simulink model "dsp_vad"  (Simulink 8.1)
settings: Solver=VariableStepDiscrete  StartTime=0.0  StopTime=count  RelTol=1e-3
PreLoadFcn:
  | % Run the setup script when the model is opened
  | setup_dsp_vad;
InitFcn:
  | % Run the setup script again just before the
  | % model is run, so that any updates made
  | % after opening are applied.
  | setup_dsp_vad;
  | %% DSPBuilder Start
  | alt_dspbuilder_update_model(bdroot)
  | %% DSPBuilder End
StartFcn:
  | %% DSPBuilder Start
  | alt_dspbuilder_hdlimport_prepare_for_simulation(bdroot)
  | %% DSPBuilder End
values from neighbouring files (symbols this model uses):
  FS = 512    [setup_dsp_vad.m]
undefined symbols (not defined in the file or in its folder): AdvDSPBDMemDisplay, dpoly, dspba, dspba_ChannelInVis, dspba_ChannelOutVis, dspba_internal_get_channel_ports, evalAionMaskParam, pow, primtype, SF, UseDontCare, value, x, y
libraries: DSPBAPrim x267, DSPBAControl x11, DspbAdvFftLibrary x10, DSPBAModelBus x7, DSPBABase x4, simulink x3, DSPBAVectorUtil x2, DSPBAUtilities x1
(part 1 of 4)
Description:
  | DSP Builder Advanced Template for Template Design implementing Primitive Subsystems
settings Model: Creator=mjervis  LastModifiedBy=AliReza
settings DebuggingCC: InheritedTsInSrcMsg=none  IntegerOverflowMsg=none
settings ConfigurationSet: Description=SimMechanics 2G

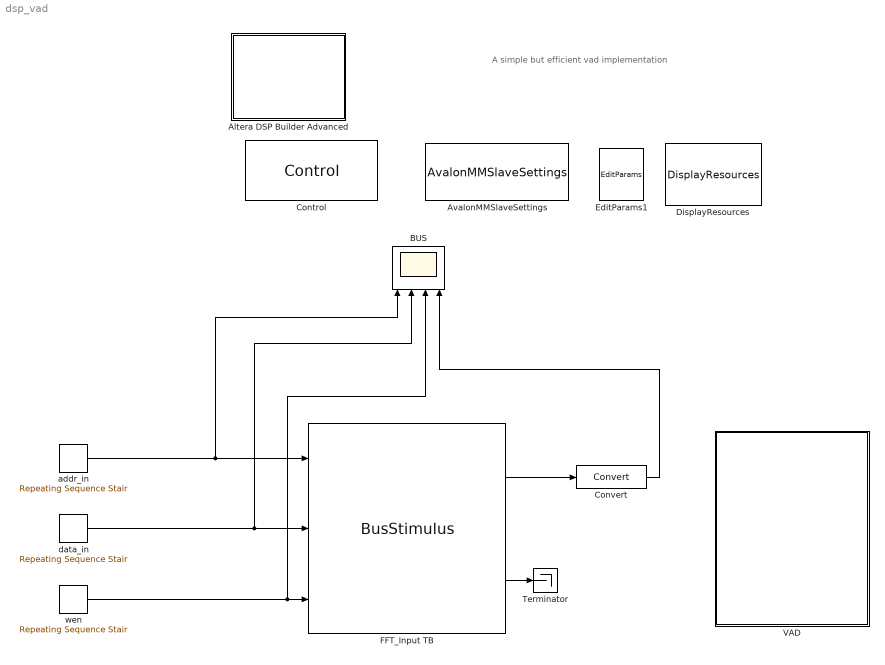
== system dsp_vad ==
  note: A simple but efficient vad implementation
  Altera DSP Builder Advanced : Subsystem  mask(DSP Builder Advanced Blockset Ignored Block){}
      settings: OpenFcn=web('http://www.altera.com', '-new');
      mask Display: image(imread('intellogo.tif'));
  AvalonMMSlaveSettings : DSPBABase/AvalonMMSlaveSettings
  BUS : Scope  NumInputPorts=4
      settings: ShowLegends=on  TimeRange=92.02958093676716  YMin=0~0~1~-1  YMax=1~1~1~1  MaxDataPoints=12290  SampleTime=auto
  "Control " : DSPBABase/Control  generate=on  language=VHDL  destination=./rtl  make_full_path=off  path_is_relative=on  autotestbench=on  signaldepth=2  coveragetestbench=off  logs=off  spacewidth=2  spacenum=1  addrwidth=10  datawidth=16  dataendian=Big Endian  hierarchicalnames=on  ramThresholdBits=-1  distRamThresholdBits=-1  mlabThresholdBits=-1  hardMultiplierThresholdLuts=-1  version=20090407  errorOnChanMismatch=1  errorOnGPIOMismatch=0  importModelsimResults=0  cycleAccurate=off  reinterpretCastMult=off  paramFile=dsp_vad_params.xml
  Convert : DSPBAPrim/Convert  primtype=convert  nInputs=1  nOutputs=1  omode=single  otype=sfix(16)  scale=2^-15  rndmethod=Biased  factor=1  satmethod=None  shift_vec=[0 1 2 -1]  value=round([0:255]/17)  inPortNames=[' '; ' ';]  outPortNames=[' '; 'c']  dspbaimage=dspba_prim.jpg  text=fprintf('convert');  style=Optimised  visibilities=8+64+256+2^17  clipdetect=off  floatPrecision=float32_m23  advOptions=[]  version=20130211
  DisplayResources : DSPBAUtilities/DisplayResources  mults=0  luts=0  memorybits=0
  EditParams1 : DSPBABase/EditParams  version=20090407
  FFT_Input TB : DSPBAModelBus/BusStimulus  SampleTime=-1  version=20140122  hasreaden=off
  Terminator : Terminator
  VAD : Subsystem
  addr_in : simulink/Sources/Repeating Sequence Stair  OutValues=dspb_vad.bus_addr_in  tsamp=1  OutMin=[]  OutMax=[]  OutDataTypeStr=fixdt(0,3)  OutputDataTypeScalingMode=Specify via dialog  OutDataType=fixdt(0,3)  ConRadixGroup=Best Precision: Vector-wise  OutScaling=[]
  data_in : simulink/Sources/Repeating Sequence Stair  OutValues=dspb_vad.bus_data_in  tsamp=1  OutMin=[]  OutMax=[]  OutDataTypeStr=single  OutputDataTypeScalingMode=single  OutDataType=fixdt(0,3)  ConRadixGroup=Best Precision: Vector-wise  OutScaling=[]
  wen : simulink/Sources/Repeating Sequence Stair  OutValues=dspb_vad.bus_wen  tsamp=1  OutMin=[]  OutMax=[]  OutDataTypeStr=fixdt('boolean')  OutputDataTypeScalingMode=Specify via dialog  OutDataType=fixdt('boolean')  ConRadixGroup=Best Precision: Vector-wise  OutScaling=[]
  wires:
  FFT_Input TB/2 -> Terminator/1
  addr_in/1 -> BUS/1, FFT_Input TB/1
  FFT_Input TB/1 -> Convert/1
  wen/1 -> BUS/3, FFT_Input TB/3
  Convert/1 -> BUS/4
  data_in/1 -> BUS/2, FFT_Input TB/2

== system dsp_vad/Altera DSP Builder Advanced ==

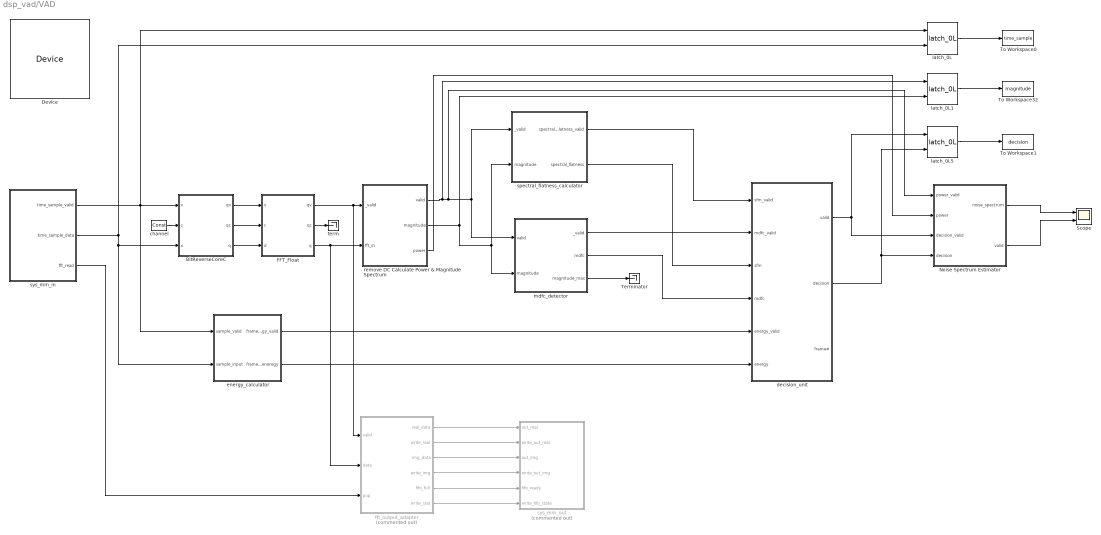
== system dsp_vad/VAD ==
  BitReverseCoreC : Subsystem  AncestorBlock=DspbAdvFftLibrary/Radix2/BitReverseCoreC  Opaque=on  mask(DSP Builder Advanced FFT Blockset){N=512, subchannels=1}
      mask prompts: N "FFT Size"; subchannels "Number of subchannels (must be a power of 2)"
      mask help: Performs bit reversal of incoming FFT frames.
      mask init:
      | block = gcb;
      | 
      | % Check that we have a legal size
      | M = ceil(log2(N));
      | if not(N == 2^M)
      |     error('%s: %d is not a power of 2', block, N);
      | end
      | 
      | % Check that we have a legal number os subchannels
      | subchannelbits = ceil(log2(subchannels));
      | if not(subchannels == 2^subchannelbits)
      |     error('%s: subchannels count %d is not a power of 2', block, N);
      | end
      | 
      | % The permutation reverses the order of the address bits
      | bitrevperm = [M-1:-1:0];
      | 
      | % Prefix permutaion with unchanging subchannel bits
      | bitrevperm = [0:subchannelbits-1,bitrevperm+subchannelbits];
      | 
      | if 1 < subchannels
      |     subchannelString = sprintf('%d subchannels',subchannels);
      | else
      |     subchannelString = '';
      | end
      mask Help: helpview(dspba.GetHelp('BitReverseCore'));
      mask Display:
      | color('w');
      | image('dspba_fft.jpg');
      | port_label('input',1,'v');
      | port_label('input',2,'c');
      | port_label('input',3,'x');
      | port_label('output',1,'qv');
      | port_label('output',2,'qc');
      | port_label('output',3,'q');
      | text(0.45,0.7,'Bit');
      | text(0.35,0.6,'Reverse');
      | text(0.40,0.5, sprintf('%d',N));
      | text(0.5,0.1,sprintf('Radix 2'),'texmode','on');
      | text(0.20,0.35,subchannelString);
  Device : DSPBABase/Device  family=Cyclone V  stratix4device=Stratix IV E  hardcopy4device=HardCopy IV E  stratix5device=Stratix V GX  device=AUTO  speed=1  stratixSpeed=-5  stratix2Speed=-3  stratix3Speed=-2  stratix4gxSpeed=-2  stratix4gtSpeed=-1  cyclone2Speed=-6  cyclone3Speed=-7  arria2Speed=-4  cyclone4eSpeed=-8  stratix5Speed=-3  arria5Speed=-4  arriaSpeed=-6  cyclone3lsSpeed=-7  cyclone5Speed=-6  arria2gzSpeed=-3  nightFurySpeed=-2  ecp2Speed=-7  hardcopycompat=off  version=20140217  max10flashmode=off  max10nomeminit=off
  FFT_Float : Subsystem  AncestorBlock=DspbAdvFftLibrary/Floating Point/FP_FFT  Opaque=on  mask{FFTstring=FFT, orderString=Bit Reversed, N=9, twiddle_type=single, faithful=false}
      mask prompts: FFTstring "FFT type"; orderString "Input Order"; N "N, where the (I)FFT has size 2^N"; twiddle_type "Data type"; faithful "Use faithful rounding"
      mask init:
      | block = gcb;
      | 
      | br_in = strcmp(orderString,'Bit Reversed');
      | IFFT = strcmp(FFTstring,'IFFT');
      | 
      | % Assume input type is the same as the twiddle type
      | data_type = dspba.namedVPFloat(twiddle_type);
      | type_strings = ...
      |     dspba.fft.full_wordgrowth(...
      |         true, false, N, data_type, data_type);
      | 
      | if br_in
      |     directionString = 'BR->NAT';
      | else
      |     directionString = 'NAT->BR';
      | end
      mask Help: helpview(dspba.GetHelp('fft'));
      mask TypeOptions FFTstring: FFT | IFFT
      mask TypeOptions orderString: Bit Reversed | Natural Order
      mask TypeOptions twiddle_type: single | double | float16_m10 | float26_m17 | float32_m23 | float35_m26 | float46_m35 | float55_m44 | float64_m52
      mask Display:
      | color('w');
      | image('dspba_fft.jpg');
      | port_label('input',1,'v');
      | port_label('input',2,'c');
      | port_label('input',3,'d');
      | port_label('output',1,'qv');
      | port_label('output',2,'qc');
      | port_label('output',3,'q');
      | text(0.30,0.65,sprintf('%s Core',FFTstring));
      | text(0.45,0.55,sprintf('2^{%d}',N),'texmode','on');
      | text(0.30,0.45,directionString);
  Noise Spectrum Estimator : Subsystem
  Scope : Scope  NumInputPorts=2
      settings: YMin=0~0  YMax=0.017~1  SaveName=ScopeData2
  Terminator : Terminator
  To Workspace0 : ToWorkspace  VariableName=time_sample  SampleTime=-1
  To Workspace1 : ToWorkspace  VariableName=decision  SampleTime=-1
  To Workspace32 : ToWorkspace  VariableName=magnitude  SampleTime=-1
  channel : DSPBAPrim/Const  primtype=const  nInputs=0  nOutputs=1  omode=Inherit via back propagation  otype=zeros(1,1,uint(8))  scale=1  rndmethod=Unbiased  factor=1  satmethod=Symmetric  shift_vec=[0 1 2 -1]  value=0  inPortNames=['+'; '+';]  outPortNames=[' ']  dspbaimage=dspba_prim.jpg  text=fprintf('%s', num2str(value));  style=Optimised  visibilities=8 + 1024  floatPrecision=float32_m23  version=20120820
  decision_unit : Subsystem
  energy_calculator : Subsystem
  fft_output_adapter : Subsystem  Commented=on
  latch_0L : DSPBAControl/latch_0L
  latch_0L1 : DSPBAControl/latch_0L
  latch_0L5 : DSPBAControl/latch_0L
  mdfc_detector : Subsystem
  remove DC Calculate Power & Magnitude Spectrum : Subsystem
  spectral_flatness_calculator : Subsystem
  sys_mm_in : Subsystem
  sys_mm_out : Subsystem  Commented=on
  "term " : Terminator
  wires:
  fft_output_adapter/1(real_data) -> sys_mm_out/1(out_real)
  fft_output_adapter/2(write_real) -> sys_mm_out/2(write_out_real)
  fft_output_adapter/3(img_data) -> sys_mm_out/3(out_img)
  fft_output_adapter/4(write_img) -> sys_mm_out/4(write_out_img)
  fft_output_adapter/5(fifo_full) -> sys_mm_out/5(fifo_ready)
  fft_output_adapter/6(write_stat) -> sys_mm_out/6(write_fifo_state)
  sys_mm_in/1(time_sample_valid) -> latch_0L/1, energy_calculator/1(sample_valid), BitReverseCoreC/1(v)
  FFT_Float/1(qv) -> remove DC Calculate Power & Magnitude Spectrum/1(_valid), fft_output_adapter/1(valid)
  FFT_Float/3(q) -> remove DC Calculate Power & Magnitude Spectrum/2(fft_in), fft_output_adapter/2(data)
  BitReverseCoreC/3(q) -> FFT_Float/3(d)
  channel/1 -> BitReverseCoreC/2(c)
  FFT_Float/2(qc) -> "term "/1
  BitReverseCoreC/2(qc) -> FFT_Float/2(c)
  BitReverseCoreC/1(qv) -> FFT_Float/1(v)
  sys_mm_in/2(time_sample_data) -> energy_calculator/2(sample_input), BitReverseCoreC/3(x), latch_0L/2
  sys_mm_in/3(fft_read) -> fft_output_adapter/3(pop)
  remove DC Calculate Power & Magnitude Spectrum/1(valid) -> spectral_flatness_calculator/1(_valid), mdfc_detector/1(valid), Noise Spectrum Estimator/1(power_valid), latch_0L1/1
  mdfc_detector/3(magnitude_max) -> Terminator/1
  energy_calculator/1(frame_energy_valid) -> decision_unit/5("energy_valid ")
  energy_calculator/2(frame_eneregy) -> decision_unit/6(energy)
  mdfc_detector/2(mdfc) -> decision_unit/4(mdfc)
  spectral_flatness_calculator/2(spectral_flatness) -> decision_unit/3(sfm)
  mdfc_detector/1(_valid) -> decision_unit/2(mdfc_valid)
  spectral_flatness_calculator/1(spectral_flatness_valid) -> decision_unit/1(sfm_valid)
  latch_0L/1 -> To Workspace0/1
  decision_unit/1(valid) -> latch_0L5/1, Noise Spectrum Estimator/3(decision_valid)
  decision_unit/2(decision) -> latch_0L5/2, Noise Spectrum Estimator/4(decision)
  latch_0L1/1 -> To Workspace32/1
  latch_0L5/1 -> To Workspace1/1
  remove DC Calculate Power & Magnitude Spectrum/2(magnitude) -> latch_0L1/2, mdfc_detector/2(magnitude), spectral_flatness_calculator/2(magnitude)
  remove DC Calculate Power & Magnitude Spectrum/3(power) -> Noise Spectrum Estimator/2(power)
  Noise Spectrum Estimator/1(noise_spectrum) -> Scope/1
  Noise Spectrum Estimator/2(valid) -> Scope/2

== system dsp_vad/VAD/BitReverseCoreC ==
  note: Bit-accurate simulation used
  note: Each block of 2^N samples should
      |  use the same channel number.
      |
      | So we latch the channel number on
      |  the last valid input (first valid output)
      | of each block.
  v : Inport
  c : Inport  Port=2
  x : Inport  Port=3
  ChannelIn : DSPBAPrim/ChannelIn  primtype=channelin  nInputs=dspba_internal_get_channel_ports(gcb)  nOutputs=dspba_internal_get_channel_ports(gcb)  omode=Inherit via internal rule  otype=sfix(16)  scale=2^-15  rndmethod=Unbiased  factor=1  satmethod=Symmetric  shift_vec=[0 1 2 -1]  value=1  inPortNames=['v'; 'c'; '0'; '1'; '2'; '3'; '4'; '5'; '6'; '7'; '8'; '9'; 'a'; 'b']  outPortNames=['v'; 'c'; '0'; '1'; '2'; '3'; '4'; '5'; '6'; '7'; '8'; '9'; 'a'; 'b']  dspbaimage=dspba_prim.jpg  text=fprintf('In');  style=Optimised  dataSignals=1  foldingEnabled=off  channels=1  sampleRate=200  packetBeginPresent=off  packetBeginEnabled=off  visibilities=1024  latencyCorrection=0  scheduleOrigin=on  version=20141013
  ChannelOut : DSPBAPrim/ChannelOut  primtype=channelout  nInputs=dspba_internal_get_channel_ports(gcb)  nOutputs=dspba_internal_get_channel_ports(gcb)  omode=Inherit via internal rule  otype=sfix(16)  scale=2^-15  rndmethod=Unbiased  factor=1  satmethod=Symmetric  shift_vec=[0 1 2 -1]  value=1  inPortNames=['v'; 'c'; '0'; '1'; '2'; '3'; '4'; '5'; '6'; '7'; '8'; '9']  outPortNames=['v'; 'c'; '0'; '1'; '2'; '3'; '4'; '5'; '6'; '7'; '8'; '9']  dspbaimage=dspba_prim.jpg  text=fprintf('Out');  style=Optimised  dataSignals=1  foldingEnabled=off  channels=1  sampleRate=200  packetBeginPresent=off  packetBeginEnabled=off  visibilities=1024  latency=0  latencyCorrection=0  version=20141013
  SynthesisInfo : DSPBAPrim/SynthesisInfo  primtype=synthinfo  nInputs=0  nOutputs=0  omode=Inherit via internal rule  otype=sfix(16)  scale=2^-15  rndmethod=Truncate  factor=1  satmethod=Symmetric  shift_vec=[0 1 2 -1]  value=99  inPortNames=[' '; ' ';]  outPortNames=[' ']  dspbaimage=dspba_prim_ctrl.jpg  text=fprintf('Style=%s', style);  style=Scheduled  visibilities=32768  constraintInUse=off  constraintRelation=>  constraintLimit=2  bitAccurate=on  version=20150220
  Transpose : DspbAdvFftLibrary/Common/Transpose  perm=bitrevperm
  latch_0L : DSPBAControl/latch_0L
  qv : Outport
  qc : Outport  Port=2
  q : Outport  Port=3
  wires:
  Transpose/3 -> latch_0L/1
  Transpose/2 -> ChannelOut/3
  Transpose/1 -> ChannelOut/1
  ChannelIn/3 -> Transpose/2
  ChannelIn/1 -> Transpose/1
  ChannelIn/2 -> latch_0L/2
  latch_0L/1 -> ChannelOut/2
  ChannelOut/3 -> q/1
  ChannelOut/2 -> qc/1
  ChannelOut/1 -> qv/1
  c/1 -> ChannelIn/2
  v/1 -> ChannelIn/1
  x/1 -> ChannelIn/3

== system dsp_vad/VAD/FFT_Float ==
  note: Bit-accurate simulation used
  note: Each block of 2^N samples should use the same channel
      | and starts arriving on the output after 2^N-1 cycles.
      |
      | So we latch the channel number on
      |  the last valid input of each block.
  v : Inport
  c : Inport  Port=2
  d : Inport  Port=3
  ChannelIn : DSPBAPrim/ChannelIn  primtype=channelin  nInputs=dspba_internal_get_channel_ports(gcb)  nOutputs=dspba_internal_get_channel_ports(gcb)  omode=Inherit via internal rule  otype=sfix(16)  scale=2^-15  rndmethod=Unbiased  factor=1  satmethod=Symmetric  shift_vec=[0 1 2 -1]  value=1  inPortNames=['v'; 'c'; '0'; '1'; '2'; '3'; '4'; '5'; '6'; '7'; '8'; '9'; 'a'; 'b']  outPortNames=['v'; 'c'; '0'; '1'; '2'; '3'; '4'; '5'; '6'; '7'; '8'; '9'; 'a'; 'b']  dspbaimage=dspba_prim.jpg  text=fprintf('In');  style=Optimised  dataSignals=1  foldingEnabled=off  channels=1  sampleRate=200  packetBeginPresent=off  packetBeginEnabled=off  visibilities=dspba_ChannelInVis(gcb)  latencyCorrection=0  scheduleOrigin=on  version=20141013
  ChannelOut1 : DSPBAPrim/ChannelOut  primtype=channelout  nInputs=dspba_internal_get_channel_ports(gcb)  nOutputs=dspba_internal_get_channel_ports(gcb)  omode=Inherit via internal rule  otype=sfix(16)  scale=2^-15  rndmethod=Unbiased  factor=1  satmethod=Symmetric  shift_vec=[0 1 2 -1]  value=1  inPortNames=['v'; 'c'; '0'; '1'; '2'; '3'; '4'; '5'; '6'; '7'; '8'; '9']  outPortNames=['v'; 'c'; '0'; '1'; '2'; '3'; '4'; '5'; '6'; '7'; '8'; '9']  dspbaimage=dspba_prim.jpg  text=fprintf('Out');  style=Optimised  dataSignals=1  foldingEnabled=off  channels=1  sampleRate=200  packetBeginPresent=off  packetBeginEnabled=off  visibilities=dspba_ChannelOutVis(gcb)  latency=0  latencyCorrection=0  version=20141013
  FP FFT Light : DspbAdvFftLibrary/Common/FFT_Light  IFFT=IFFT  subchannels=1  br_in=br_in  N=N  in_type=data_type  type_strings=type_strings  faithful=faithful  wirecount=1
  SynthesisInfo : DSPBAPrim/SynthesisInfo  primtype=synthinfo  nInputs=0  nOutputs=0  omode=Inherit via internal rule  otype=sfix(16)  scale=2^-15  rndmethod=Truncate  factor=1  satmethod=Symmetric  shift_vec=[0 1 2 -1]  value=99  inPortNames=[' '; ' ';]  outPortNames=[' ']  dspbaimage=dspba_prim.jpg  text=fprintf('Style=%s', style);  style=Scheduled  visibilities=32768  constraintInUse=off  constraintRelation=>  constraintLimit=2  bitAccurate=on  version=20150220
  latch_0L : DSPBAControl/latch_0L
  qv : Outport
  qc : Outport  Port=2
  q : Outport  Port=3
  wires:
  FP FFT Light/3 -> latch_0L/1
  ChannelIn/2 -> latch_0L/2
  FP FFT Light/2 -> ChannelOut1/3
  ChannelIn/3 -> FP FFT Light/2
  v/1 -> ChannelIn/1
  d/1 -> ChannelIn/3
  c/1 -> ChannelIn/2
  ChannelIn/1 -> FP FFT Light/1
  latch_0L/1 -> ChannelOut1/2
  ChannelOut1/3 -> q/1
  ChannelOut1/1 -> qv/1
  ChannelOut1/2 -> qc/1
  FP FFT Light/1 -> ChannelOut1/1

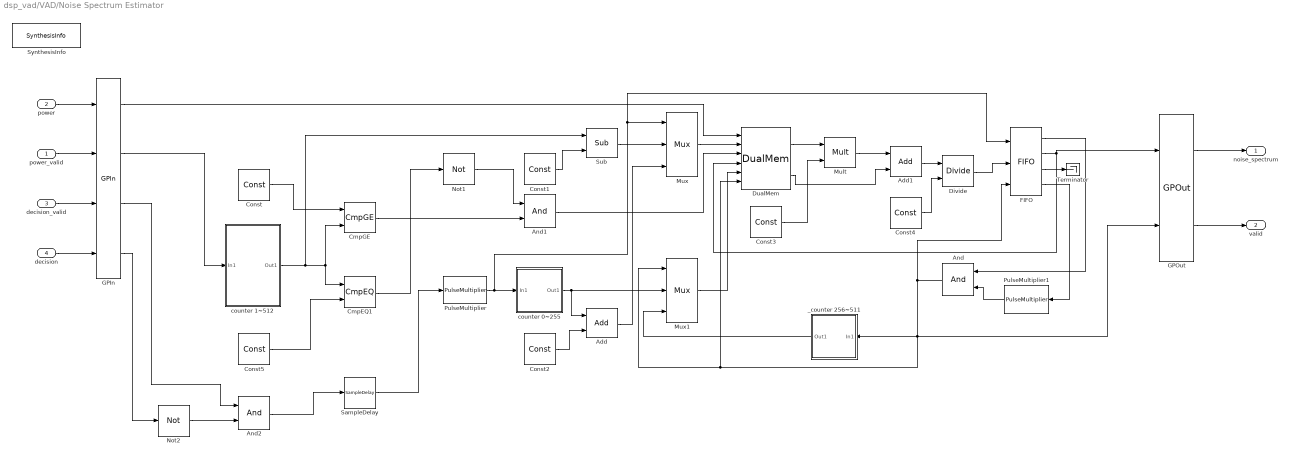
== system dsp_vad/VAD/Noise Spectrum Estimator ==
  power_valid : Inport
  power : Inport  Port=2
  decision_valid : Inport  Port=3
  decision : Inport  Port=4
  Add : DSPBAPrim/Add  primtype=add  nInputs=evalAionMaskParam(gcb,'value',1)  nOutputs=1  omode=Specify via dialog  otype=ufix(10)  scale=2^-0  rndmethod=Unbiased  factor=1  satmethod=Symmetric  shift_vec=[0 1 2 -1]  value=2  inPortNames=[' '; ' ';]  outPortNames=[' ']  dspbaimage=dspba_prim.jpg  text=fprintf('+');  style=Optimised  visibilities=1032+2^17+2^18+2^19  genFPC=off  floatRounding=correct  advOptions=[]  version=20130821
  Add1 : DSPBAPrim/Add  primtype=add  nInputs=evalAionMaskParam(gcb,'value',1)  nOutputs=1  omode=Inherit via internal rule  otype=ufix(10)  scale=2^-0  rndmethod=Unbiased  factor=1  satmethod=Symmetric  shift_vec=[0 1 2 -1]  value=2  inPortNames=[' '; ' ';]  outPortNames=[' ']  dspbaimage=dspba_prim.jpg  text=fprintf('+');  style=Optimised  visibilities=1032+2^17+2^18+2^19  genFPC=off  floatRounding=correct  advOptions=[]  version=20130821
  And : DSPBAPrim/And  primtype=and  nInputs=2  nOutputs=1  omode=Inherit via internal rule  otype=sfix(16)  scale=2^-15  rndmethod=Unbiased  factor=1  satmethod=Symmetric  shift_vec=[0 1 2 -1]  value=0  inPortNames=[' '; ' '; ' '; ' '; ' '; ' '; ' '; ' '; ' '; ' '; ' '; ' '; ' '; ' '; ' '; ' '; ]  outPortNames=[' ']  dspbaimage=dspba_prim.jpg  text=fprintf('&');  style=Optimised  visibilities=8+2  version=20090407
  And1 : DSPBAPrim/And  primtype=and  nInputs=2  nOutputs=1  omode=Inherit via internal rule  otype=sfix(16)  scale=2^-15  rndmethod=Unbiased  factor=1  satmethod=Symmetric  shift_vec=[0 1 2 -1]  value=0  inPortNames=[' '; ' '; ' '; ' '; ' '; ' '; ' '; ' '; ' '; ' '; ' '; ' '; ' '; ' '; ' '; ' '; ]  outPortNames=[' ']  dspbaimage=dspba_prim.jpg  text=fprintf('&');  style=Optimised  visibilities=8+2  version=20090407
  And2 : DSPBAPrim/And  primtype=and  nInputs=2  nOutputs=1  omode=Inherit via internal rule  otype=sfix(16)  scale=2^-15  rndmethod=Unbiased  factor=1  satmethod=Symmetric  shift_vec=[0 1 2 -1]  value=0  inPortNames=[' '; ' '; ' '; ' '; ' '; ' '; ' '; ' '; ' '; ' '; ' '; ' '; ' '; ' '; ' '; ' '; ]  outPortNames=[' ']  dspbaimage=dspba_prim.jpg  text=fprintf('&');  style=Optimised  visibilities=8+2  version=20090407
  CmpEQ1 : DSPBAPrim/CmpEQ  primtype=cmpeq  nInputs=2  nOutputs=1  omode=boolean  otype=sfix(16)  scale=2^-15  rndmethod=Unbiased  factor=1  satmethod=Symmetric  shift_vec=[0 1 2 -1]  value=0  inPortNames=[' '; ' ';]  outPortNames=[' ']  dspbaimage=dspba_prim.jpg  text=fprintf('==');  style=Optimised  visibilities=0  advOptions=[]  version=20130117
  CmpGE : DSPBAPrim/CmpGE  primtype=cmpgte  nInputs=2  nOutputs=1  omode=boolean  otype=sfix(16)  scale=2^-15  rndmethod=Unbiased  factor=1  satmethod=Symmetric  shift_vec=[0 1 2 -1]  value=0  inPortNames=['a'; 'b';]  outPortNames=[' ']  dspbaimage=dspba_prim.jpg  text=fprintf('a>=b');  style=Optimised  visibilities=0  advOptions=[]  version=20130117
  Const : DSPBAPrim/Const  primtype=const  nInputs=0  nOutputs=1  omode=Specify via dialog  otype=ufix(9)  scale=2^-0  rndmethod=Unbiased  factor=1  satmethod=Symmetric  shift_vec=[0 1 2 -1]  value=256  inPortNames=['+'; '+';]  outPortNames=[' ']  dspbaimage=dspba_prim.jpg  text=fprintf('%s', num2str(value));  style=Optimised  visibilities=8 + 1024  floatPrecision=float32_m23  version=20120820
  Const1 : DSPBAPrim/Const  primtype=const  nInputs=0  nOutputs=1  omode=Specify via dialog  otype=ufix(10)  scale=2^-0  rndmethod=Unbiased  factor=1  satmethod=Symmetric  shift_vec=[0 1 2 -1]  value=1  inPortNames=['+'; '+';]  outPortNames=[' ']  dspbaimage=dspba_prim.jpg  text=fprintf('%s', num2str(value));  style=Optimised  visibilities=8 + 1024  floatPrecision=float32_m23  version=20120820
  Const2 : DSPBAPrim/Const  primtype=const  nInputs=0  nOutputs=1  omode=Specify via dialog  otype=ufix(10)  scale=2^-0  rndmethod=Unbiased  factor=1  satmethod=Symmetric  shift_vec=[0 1 2 -1]  value=256  inPortNames=['+'; '+';]  outPortNames=[' ']  dspbaimage=dspba_prim.jpg  text=fprintf('%s', num2str(value));  style=Optimised  visibilities=8 + 1024  floatPrecision=float32_m23  version=20120820
  Const3 : DSPBAPrim/Const  primtype=const  nInputs=0  nOutputs=1  omode=single  otype=sfix(16)  scale=2^-15  rndmethod=Unbiased  factor=1  satmethod=Symmetric  shift_vec=[0 1 2 -1]  value=30  inPortNames=['+'; '+';]  outPortNames=[' ']  dspbaimage=dspba_prim.jpg  text=fprintf('%s', num2str(value));  style=Optimised  visibilities=8 + 1024  floatPrecision=float32_m23  version=20120820
  Const4 : DSPBAPrim/Const  primtype=const  nInputs=0  nOutputs=1  omode=single  otype=sfix(16)  scale=2^-15  rndmethod=Unbiased  factor=1  satmethod=Symmetric  shift_vec=[0 1 2 -1]  value=31  inPortNames=['+'; '+';]  outPortNames=[' ']  dspbaimage=dspba_prim.jpg  text=fprintf('%s', num2str(value));  style=Optimised  visibilities=8 + 1024  floatPrecision=float32_m23  version=20120820
  Const5 : DSPBAPrim/Const  primtype=const  nInputs=0  nOutputs=1  omode=Specify via dialog  otype=ufix(10)  scale=2^-0  rndmethod=Unbiased  factor=1  satmethod=Symmetric  shift_vec=[0 1 2 -1]  value=0  inPortNames=['+'; '+';]  outPortNames=[' ']  dspbaimage=dspba_prim.jpg  text=fprintf('%s', num2str(value));  style=Optimised  visibilities=8 + 1024  floatPrecision=float32_m23  version=20120820
  Divide : DSPBAPrim/Divide  primtype=divide  nInputs=2  nOutputs=1  omode=Inherit via internal rule  otype=sfix(16)  scale=2^-15  rndmethod=Unbiased  factor=1  satmethod=Symmetric  shift_vec=[0 1 2 -1]  value=round([0:255]/17)  inPortNames=[' '; ' ';]  outPortNames=[' ']  dspbaimage=dspba_prim.jpg  text=fprintf('a\n----\nb');  style=Optimised  visibilities=8+2^17+2^18  floatRounding=correct  advOptions=[]  version=20130115
  DualMem : DSPBAPrim/DualMem  primtype=dualmem  nInputs=6  nOutputs=2  omode=single  otype=sfix(16)  scale=2^-15  rndmethod=Unbiased  factor=1  satmethod=Symmetric  shift_vec=[0 1 2 -1]  value=[zeros(512, 1)]  inPortNames=['d1'; 'a1'; 'w1'; 'd2'; 'a2'; 'w2']  outPortNames=['q1'; 'q2']  dspbaimage=dspba_prim.jpg  text=fprintf('dmem%s',AdvDSPBDMemDisplay(UseDontCare));  style=Optimised  visibilities=8 + 1024 + 2^17 + 2^18  UseDontCare=on  TwinWritePorts=on  version=20141001
  FIFO : DSPBAPrim/FIFO  primtype=fifo  nInputs=3  nOutputs=4  omode=Inherit via internal rule  otype=sfix(16)  scale=2^-15  rndmethod=Unbiased  factor=1  satmethod=Symmetric  shift_vec=[0 1 2 -1]  value=[256 1 256]  inPortNames=['w'; 'd'; 'r'; 'f']  outPortNames=['v'; 'q'; 't'; 'f']  dspbaimage=dspba_prim.jpg  text=fprintf('fifo');  style=Optimised  visibilities=263168  version=20130808  user_sclr=off
  GPIn : DSPBAPrim/GPIn  primtype=gpin  nInputs=evalAionMaskParam(gcb,'value',1)  nOutputs=evalAionMaskParam(gcb,'value',1)  omode=Inherit via internal rule  otype=sfix(16)  scale=2^-15  rndmethod=Unbiased  factor=1  satmethod=Symmetric  shift_vec=[0 1 2 -1]  value=4  inPortNames=[' ' ' ' ' ' ' ' ' ' ' ' ' ' ' ' ' ' ' ' ' ' ' ' ' ' ' ' ' ' ' ' ' ' ' ' ' ' ' ' ' ' ' ' ' ' ' ' ' ' ' ' ' ' ' ' ' ' ' ' ' ' ' ' ' ' ' ' ' ']'  outPortNames=[' ' ' ' ' ' ' ' ' ' ' ' ' ' ' ' ' ' ' ' ' ' ' ' ' ' ' ' ' ' ' ' ' ' ' ' ' ' ' ' ' ' ' ' ' ' ' ' ' ' ' ' ' ' ' ' ' ' ' ' ' ' ' ' ' ' ' ' ' ']'  dspbaimage=dspba_prim.jpg  text=fprintf('GPIn');  style=Optimised  visibilities=1024  latencyCorrection=0  scheduleOrigin=on  version=20090407
  GPOut : DSPBAPrim/GPOut  primtype=gpout  nInputs=evalAionMaskParam(gcb,'value',1)  nOutputs=evalAionMaskParam(gcb,'value',1)  omode=Inherit via internal rule  otype=sfix(16)  scale=2^-15  rndmethod=Unbiased  factor=1  satmethod=Symmetric  shift_vec=[0 1 2 -1]  value=2  inPortNames=[' ' ' ' ' ' ' ' ' ' ' ' ' ' ' ' ' ' ' ' ' ' ' ' ' ' ' ' ' ' ' ' ' ' ' ' ' ' ' ' ' ' ' ' ' ' ' ' ' ' ' ' ' ' ' ' ' ' ' ' ' ' ' ' ' ' ' ' ' ']'  outPortNames=[' ' ' ' ' ' ' ' ' ' ' ' ' ' ' ' ' ' ' ' ' ' ' ' ' ' ' ' ' ' ' ' ' ' ' ' ' ' ' ' ' ' ' ' ' ' ' ' ' ' ' ' ' ' ' ' ' ' ' ' ' ' ' ' ' ' ' ' ' ']'  dspbaimage=dspba_prim.jpg  text=fprintf('GPOut');  style=Optimised  visibilities=1024  latencyCorrection=0  version=20090407
  Mult : DSPBAPrim/Mult  primtype=mult  nInputs=2  nOutputs=1  omode=Inherit via internal rule  otype=sfix(16)  scale=2^-15  rndmethod=Unbiased  factor=1  satmethod=Symmetric  shift_vec=[0 1 2 -1]  value=0  inPortNames=[' '; ' ';]  outPortNames=[' ']  dspbaimage=dspba_prim.jpg  text=fprintf('X');  style=Optimised  visibilities=8+2^18+2^19  floatPrecision=float32_m23  floatRounding=correct  advOptions=[]  version=20130115
  Mux : DSPBAPrim/Mux  primtype=mux  nInputs=evalAionMaskParam(gcb,'value',1)+1  nOutputs=1  omode=Inherit via internal rule  otype=sfix(16)  scale=2^-15  rndmethod=Unbiased  factor=1  satmethod=Symmetric  shift_vec=[0 1 2 -1]  value=2  inPortNames=['s '; 'd0'; 'd1'; 'd2'; 'd3'; 'd4'; 'd5'; 'd6'; 'd7'; 'd8'; 'd9';]  outPortNames=[' ']  dspbaimage=dspba_prim.jpg  text=fprintf('%s', primtype);  style=Optimised  visibilities=1032  version=20131025
  Mux1 : DSPBAPrim/Mux  primtype=mux  nInputs=evalAionMaskParam(gcb,'value',1)+1  nOutputs=1  omode=Inherit via internal rule  otype=sfix(16)  scale=2^-15  rndmethod=Unbiased  factor=1  satmethod=Symmetric  shift_vec=[0 1 2 -1]  value=2  inPortNames=['s '; 'd0'; 'd1'; 'd2'; 'd3'; 'd4'; 'd5'; 'd6'; 'd7'; 'd8'; 'd9';]  outPortNames=[' ']  dspbaimage=dspba_prim.jpg  text=fprintf('%s', primtype);  style=Optimised  visibilities=1032  version=20131025
  Not1 : DSPBAPrim/Not  primtype=not  nInputs=1  nOutputs=1  omode=Inherit via internal rule  otype=sfix(16)  scale=2^-15  rndmethod=Unbiased  factor=1  satmethod=Symmetric  shift_vec=[0 1 2 -1]  value=0  inPortNames=[' '; ' ';]  outPortNames=[' ']  dspbaimage=dspba_prim.jpg  text=fprintf('~');  style=Optimised  visibilities=8  version=20090407
  Not2 : DSPBAPrim/Not  primtype=not  nInputs=1  nOutputs=1  omode=Inherit via internal rule  otype=sfix(16)  scale=2^-15  rndmethod=Unbiased  factor=1  satmethod=Symmetric  shift_vec=[0 1 2 -1]  value=0  inPortNames=[' '; ' ';]  outPortNames=[' ']  dspbaimage=dspba_prim.jpg  text=fprintf('~');  style=Optimised  visibilities=8  version=20090407
  PulseMultiplier : DspbAdvFftLibrary/Common/PulseMultiplier  N=8
  PulseMultiplier1 : DspbAdvFftLibrary/Common/PulseMultiplier  N=8
  SampleDelay : DSPBAPrim/SampleDelay  primtype=sampdelay  nInputs=1  nOutputs=1  omode=Inherit via internal rule  otype=sfix(16)  scale=2^-15  rndmethod=Unbiased  factor=1  satmethod=Symmetric  shift_vec=[0 1 2 -1]  value=1  inPortNames=[' '; ' ';]  outPortNames=[' ']  dspbaimage=dspba_prim.jpg  text=dpoly(1, eye(1,value+1), 'z')  style=Optimised  visibilities=8 + 1024 + 2^17 + 2^18  flexible=off  slackgroup=0  augmented=0  version=20090407  advOptions=[]
  Sub : DSPBAPrim/Sub  primtype=sub  nInputs=2  nOutputs=1  omode=Specify via dialog  otype=ufix(10)  scale=2^-0  rndmethod=Unbiased  factor=1  satmethod=Symmetric  shift_vec=[0 1 2 -1]  value=0  inPortNames=['+'; '-';]  outPortNames=[' ']  dspbaimage=dspba_prim.jpg  text=fprintf('-');  style=Optimised  visibilities=8+2^17+2^18  floatRounding=correct  advOptions=[]  version=20130115
  SynthesisInfo : DSPBAPrim/SynthesisInfo  primtype=synthinfo  nInputs=0  nOutputs=0  omode=Inherit via internal rule  otype=sfix(16)  scale=2^-15  rndmethod=Truncate  factor=1  satmethod=Symmetric  shift_vec=[0 1 2 -1]  value=99  inPortNames=[' '; ' ';]  outPortNames=[' ']  dspbaimage=dspba_prim_ctrl.jpg  text=fprintf('Style=%s', style);  style=Scheduled  visibilities=2^17+2^18+2^19+2^20  constraintInUse=off  constraintRelation=>  constraintLimit=2  bitAccurate=off  version=20150220
  Terminator : Terminator
  _counter 256~511 : Subsystem
  counter 0~255 : Subsystem
  counter 1~512 : Subsystem
  noise_spectrum : Outport
  valid : Outport  Port=2
  wires:
  CmpGE/1 -> And1/2
  Const/1 -> CmpGE/1
  Not1/1 -> And1/1
  power/1 -> GPIn/1
  power_valid/1 -> GPIn/2
  decision_valid/1 -> GPIn/3
  decision/1 -> GPIn/4
  GPIn/3 -> And2/1
  GPIn/4 -> Not2/1
  Not2/1 -> And2/2
  GPIn/2 -> counter 1~512/1(In1)
  counter 1~512/1(Out1) -> Sub/1, CmpGE/2, CmpEQ1/1
  Const5/1 -> CmpEQ1/2
  And1/1 -> DualMem/3
  Const1/1 -> Sub/2
  CmpEQ1/1 -> Not1/1
  GPIn/1 -> DualMem/1
  PulseMultiplier/1 -> counter 0~255/1(In1), FIFO/1, Mux/1
  Sub/1 -> Mux/2
  Mux/1 -> DualMem/2
  counter 0~255/1(Out1) -> Add/1, Mux1/2
  Const2/1 -> Add/2
  Add/1 -> Mux/3
  And2/1 -> SampleDelay/1
  SampleDelay/1 -> PulseMultiplier/1
  FIFO/1 -> And/1
  PulseMultiplier1/1 -> And/2
  FIFO/4 -> PulseMultiplier1/1
  FIFO/2 -> GPOut/1, DualMem/4
  And/1 -> DualMem/6, Mux1/1, _counter 256~511/1(In1), GPOut/2, FIFO/3
  Mux1/1 -> DualMem/5
  _counter 256~511/1(Out1) -> Mux1/3
  Divide/1 -> FIFO/2
  Add1/1 -> Divide/1
  Const4/1 -> Divide/2
  DualMem/1 -> Mult/1
  Mult/1 -> Add1/1
  Const3/1 -> Mult/2
  DualMem/2 -> Add1/2
  FIFO/3 -> Terminator/1
  GPOut/2 -> valid/1
  GPOut/1 -> noise_spectrum/1

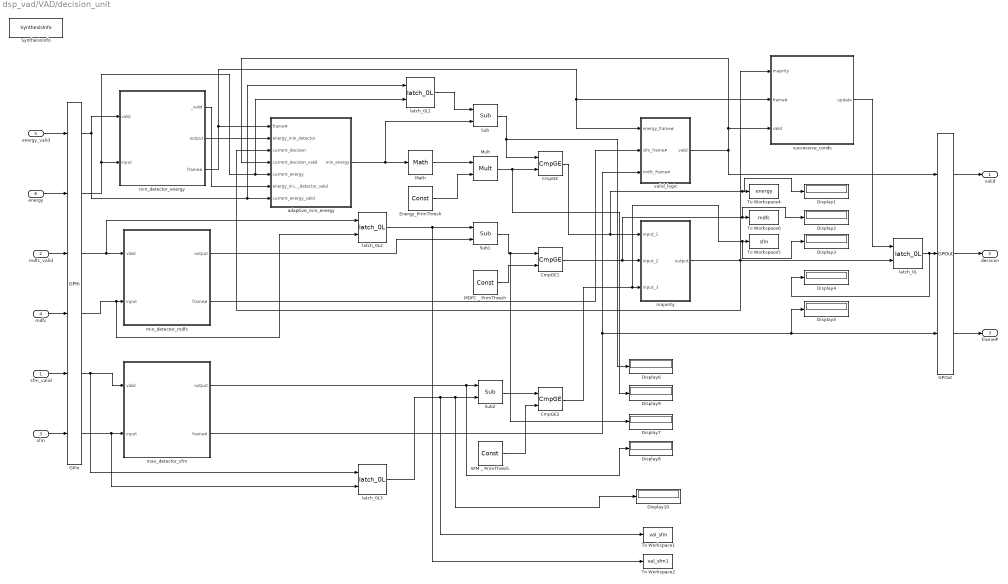
== system dsp_vad/VAD/decision_unit ==
  sfm_valid : Inport
  mdfc_valid : Inport  Port=2
  sfm : Inport  Port=3
  mdfc : Inport  Port=4
  "energy_valid " : Inport  Port=5
  energy : Inport  Port=6
  CmpGE : DSPBAPrim/CmpGE  primtype=cmpgte  nInputs=2  nOutputs=1  omode=boolean  otype=sfix(16)  scale=2^-15  rndmethod=Unbiased  factor=1  satmethod=Symmetric  shift_vec=[0 1 2 -1]  value=0  inPortNames=['a'; 'b';]  outPortNames=[' ']  dspbaimage=dspba_prim.jpg  text=fprintf('a>=b');  style=Optimised  visibilities=0  advOptions=[]  version=20130117
  CmpGE1 : DSPBAPrim/CmpGE  primtype=cmpgte  nInputs=2  nOutputs=1  omode=boolean  otype=sfix(16)  scale=2^-15  rndmethod=Unbiased  factor=1  satmethod=Symmetric  shift_vec=[0 1 2 -1]  value=0  inPortNames=['a'; 'b';]  outPortNames=[' ']  dspbaimage=dspba_prim.jpg  text=fprintf('a>=b');  style=Optimised  visibilities=0  advOptions=[]  version=20130117
  CmpGE2 : DSPBAPrim/CmpGE  primtype=cmpgte  nInputs=2  nOutputs=1  omode=boolean  otype=sfix(16)  scale=2^-15  rndmethod=Unbiased  factor=1  satmethod=Symmetric  shift_vec=[0 1 2 -1]  value=0  inPortNames=['a'; 'b';]  outPortNames=[' ']  dspbaimage=dspba_prim.jpg  text=fprintf('a>=b');  style=Optimised  visibilities=0  advOptions=[]  version=20130117
  Display{1..10} (10 alike) : Display
  Energy_PrimThresh : DSPBAPrim/Const  primtype=const  nInputs=0  nOutputs=1  omode=single  otype=sfix(16)  scale=2^-15  rndmethod=Unbiased  factor=1  satmethod=Symmetric  shift_vec=[0 1 2 -1]  value=-0.008  inPortNames=['+'; '+';]  outPortNames=[' ']  dspbaimage=dspba_prim.jpg  text=fprintf('%s', num2str(value));  style=Optimised  visibilities=8 + 1024  floatPrecision=float32_m23  version=20120820
  GPIn : DSPBAPrim/GPIn  primtype=gpin  nInputs=evalAionMaskParam(gcb,'value',1)  nOutputs=evalAionMaskParam(gcb,'value',1)  omode=Inherit via internal rule  otype=sfix(16)  scale=2^-15  rndmethod=Unbiased  factor=1  satmethod=Symmetric  shift_vec=[0 1 2 -1]  value=6  inPortNames=[' ' ' ' ' ' ' ' ' ' ' ' ' ' ' ' ' ' ' ' ' ' ' ' ' ' ' ' ' ' ' ' ' ' ' ' ' ' ' ' ' ' ' ' ' ' ' ' ' ' ' ' ' ' ' ' ' ' ' ' ' ' ' ' ' ' ' ' ' ']'  outPortNames=[' ' ' ' ' ' ' ' ' ' ' ' ' ' ' ' ' ' ' ' ' ' ' ' ' ' ' ' ' ' ' ' ' ' ' ' ' ' ' ' ' ' ' ' ' ' ' ' ' ' ' ' ' ' ' ' ' ' ' ' ' ' ' ' ' ' ' ' ' ']'  dspbaimage=dspba_prim.jpg  text=fprintf('GPIn');  style=Optimised  visibilities=1024  latencyCorrection=0  scheduleOrigin=on  version=20090407
  GPOut : DSPBAPrim/GPOut  primtype=gpout  nInputs=evalAionMaskParam(gcb,'value',1)  nOutputs=evalAionMaskParam(gcb,'value',1)  omode=Inherit via internal rule  otype=sfix(16)  scale=2^-15  rndmethod=Unbiased  factor=1  satmethod=Symmetric  shift_vec=[0 1 2 -1]  value=3  inPortNames=[' ' ' ' ' ' ' ' ' ' ' ' ' ' ' ' ' ' ' ' ' ' ' ' ' ' ' ' ' ' ' ' ' ' ' ' ' ' ' ' ' ' ' ' ' ' ' ' ' ' ' ' ' ' ' ' ' ' ' ' ' ' ' ' ' ' ' ' ' ']'  outPortNames=[' ' ' ' ' ' ' ' ' ' ' ' ' ' ' ' ' ' ' ' ' ' ' ' ' ' ' ' ' ' ' ' ' ' ' ' ' ' ' ' ' ' ' ' ' ' ' ' ' ' ' ' ' ' ' ' ' ' ' ' ' ' ' ' ' ' ' ' ' ']'  dspbaimage=dspba_prim.jpg  text=fprintf('GPOut');  style=Optimised  visibilities=1024  latencyCorrection=0  version=20090407
  MDFC _ PrimThresh : DSPBAPrim/Const  primtype=const  nInputs=0  nOutputs=1  omode=single  otype=sfix(16)  scale=2^-15  rndmethod=Unbiased  factor=1  satmethod=Symmetric  shift_vec=[0 1 2 -1]  value=155  inPortNames=['+'; '+';]  outPortNames=[' ']  dspbaimage=dspba_prim.jpg  text=fprintf('%s', num2str(value));  style=Optimised  visibilities=8 + 1024  floatPrecision=float32_m23  version=20120820
  Math : DSPBAPrim/Math  primtype=mathfunc  nInputs=1  nOutputs=1  omode=Inherit via internal rule  otype=sfix(16)  scale=2^-15  rndmethod=Unbiased  factor=1  satmethod=Symmetric  shift_vec=[0 1 2 -1]  value=round([0:255]/17)  inPortNames=[' '; ' ';]  outPortNames=[' ']  dspbaimage=dspba_prim_float.jpg  text=fprintf('exp(x)');  style=Optimised  visibilities=2^17  functionExpr=log10(x)  advOptions=[]  floatRounding=correct  version=20130910
  Mult : DSPBAPrim/Mult  primtype=mult  nInputs=2  nOutputs=1  omode=Inherit via internal rule  otype=sfix(16)  scale=2^-15  rndmethod=Unbiased  factor=1  satmethod=Symmetric  shift_vec=[0 1 2 -1]  value=0  inPortNames=[' '; ' ';]  outPortNames=[' ']  dspbaimage=dspba_prim.jpg  text=fprintf('X');  style=Optimised  visibilities=8+2^18+2^19  floatPrecision=float32_m23  floatRounding=correct  advOptions=[]  version=20130115
  SFM _ PrimThresh : DSPBAPrim/Const  primtype=const  nInputs=0  nOutputs=1  omode=single  otype=sfix(16)  scale=2^-15  rndmethod=Unbiased  factor=1  satmethod=Symmetric  shift_vec=[0 1 2 -1]  value=2  inPortNames=['+'; '+';]  outPortNames=[' ']  dspbaimage=dspba_prim.jpg  text=fprintf('%s', num2str(value));  style=Optimised  visibilities=8 + 1024  floatPrecision=float32_m23  version=20120820
  Sub : DSPBAPrim/Sub  primtype=sub  nInputs=2  nOutputs=1  omode=Inherit via internal rule with word growth  otype=sfix(16)  scale=2^-15  rndmethod=Unbiased  factor=1  satmethod=Symmetric  shift_vec=[0 1 2 -1]  value=0  inPortNames=['+'; '-';]  outPortNames=[' ']  dspbaimage=dspba_prim.jpg  text=fprintf('-');  style=Optimised  visibilities=8+2^17+2^18  floatRounding=correct  advOptions=[]  version=20130115
  Sub1 : DSPBAPrim/Sub  primtype=sub  nInputs=2  nOutputs=1  omode=Inherit via internal rule with word growth  otype=sfix(16)  scale=2^-15  rndmethod=Unbiased  factor=1  satmethod=Symmetric  shift_vec=[0 1 2 -1]  value=0  inPortNames=['+'; '-';]  outPortNames=[' ']  dspbaimage=dspba_prim.jpg  text=fprintf('-');  style=Optimised  visibilities=8+2^17+2^18  floatRounding=correct  advOptions=[]  version=20130115
  Sub2 : DSPBAPrim/Sub  primtype=sub  nInputs=2  nOutputs=1  omode=Inherit via internal rule with word growth  otype=sfix(16)  scale=2^-15  rndmethod=Unbiased  factor=1  satmethod=Symmetric  shift_vec=[0 1 2 -1]  value=0  inPortNames=['+'; '-';]  outPortNames=[' ']  dspbaimage=dspba_prim.jpg  text=fprintf('-');  style=Optimised  visibilities=8+2^17+2^18  floatRounding=correct  advOptions=[]  version=20130115
  SynthesisInfo : DSPBAPrim/SynthesisInfo  primtype=synthinfo  nInputs=0  nOutputs=0  omode=Inherit via internal rule  otype=sfix(16)  scale=2^-15  rndmethod=Truncate  factor=1  satmethod=Symmetric  shift_vec=[0 1 2 -1]  value=99  inPortNames=[' '; ' ';]  outPortNames=[' ']  dspbaimage=dspba_prim_ctrl.jpg  text=fprintf('Style=%s', style);  style=Scheduled  visibilities=2^17+2^18+2^19+2^20  constraintInUse=off  constraintRelation=>  constraintLimit=2  bitAccurate=on  version=20150220
  To Workspace1 : ToWorkspace  VariableName=val_sfm  SampleTime=-1
  To Workspace2 : ToWorkspace  VariableName=val_sfm1  SampleTime=-1
  To Workspace4 : ToWorkspace  VariableName=energy  SampleTime=-1
  To Workspace5 : ToWorkspace  VariableName=sfm  SampleTime=-1
  To Workspace6 : ToWorkspace  VariableName=mdfc  SampleTime=-1
  adaptive_min_energy : Subsystem
  latch_0L{,1..3} (4 alike) : DSPBAControl/latch_0L
  majority : Subsystem
  max_detector_sfm : Subsystem
  min_detector_energy : Subsystem
  min_detector_mdfc : Subsystem
  successive_conds : Subsystem
  valid_logic : Subsystem
  valid : Outport
  decision : Outport  Port=2
  frame# : Outport  Port=3
  wires:
  mdfc_valid/1 -> GPIn/3
  "energy_valid "/1 -> GPIn/1
  energy/1 -> GPIn/2
  GPIn/1 -> min_detector_energy/1(valid), latch_0L1/1, adaptive_min_energy/7(current_energy_valid)
  GPIn/3 -> latch_0L2/1, min_detector_mdfc/1(valid)
  GPIn/4 -> latch_0L2/2, min_detector_mdfc/2(input)
  sfm_valid/1 -> GPIn/5
  GPIn/5 -> max_detector_sfm/1(valid), latch_0L3/1
  sfm/1 -> GPIn/6
  GPIn/6 -> latch_0L3/2, max_detector_sfm/2(input)
  mdfc/1 -> GPIn/4
  Sub/1 -> Display6/1, CmpGE/1
  min_detector_mdfc/1(output) -> Sub1/2
  MDFC _ PrimThresh/1 -> CmpGE1/2
  Sub1/1 -> Display7/1, CmpGE1/1
  Sub2/1 -> CmpGE2/1
  GPOut/2 -> decision/1
  GPOut/3 -> frame#/1
  min_detector_mdfc/2(frame#) -> valid_logic/2(sfm_frame#)
  min_detector_energy/3(frame#) -> valid_logic/1(energy_frame#), successive_conds/2(frame#), adaptive_min_energy/1(frame#)
  max_detector_sfm/2(frame#) -> Display5/1, GPOut/3, valid_logic/3(mdfc_frame#)
  GPOut/1 -> valid/1
  Math/1 -> Mult/1
  min_detector_energy/2(output) -> adaptive_min_energy/2(energy_min_detector)
  min_detector_energy/1(_valid) -> adaptive_min_energy/6(energy_min_detector_valid)
  adaptive_min_energy/1(min_energy) -> Sub/2, Math/1
  Energy_PrimThresh/1 -> Mult/2
  majority/1(output) -> adaptive_min_energy/3(current_decision), successive_conds/1(majority), latch_0L/2
  successive_conds/1(update) -> latch_0L/1
  valid_logic/1(valid) -> adaptive_min_energy/4(current_decision_valid), successive_conds/3(valid), GPOut/1
  latch_0L/1 -> Display4/1, GPOut/2
  CmpGE1/1 -> Display2/1, To Workspace6/1, majority/2(input_2)
  CmpGE2/1 -> Display3/1, To Workspace5/1, majority/3(input_3)
  Mult/1 -> Display9/1, CmpGE/2
  SFM _ PrimThresh/1 -> CmpGE2/2
  CmpGE/1 -> Display1/1, To Workspace4/1, majority/1(input_1)
  latch_0L1/1 -> Sub/1
  GPIn/2 -> min_detector_energy/2(input), latch_0L1/2, adaptive_min_energy/5(current_energy)
  latch_0L3/1 -> To Workspace1/1, Display10/1, Sub2/2
  max_detector_sfm/1(output) -> Display8/1, Sub2/1
  latch_0L2/1 -> To Workspace2/1, Sub1/1

== system dsp_vad/VAD/energy_calculator ==
  sample_valid : Inport
  sample_input : Inport  Port=2
  Const : DSPBAPrim/Const  primtype=const  nInputs=0  nOutputs=1  omode=single  otype=fixdt(0,2)  scale=1  rndmethod=Unbiased  factor=1  satmethod=Symmetric  shift_vec=[0 1 2 -1]  value=2  inPortNames=['+'; '+';]  outPortNames=[' ']  dspbaimage=dspba_prim.jpg  text=fprintf('%s', num2str(value));  style=Optimised  visibilities=8 + 1024  floatPrecision=float32_m23  version=20120820
  GPIn : DSPBAPrim/GPIn  primtype=gpin  nInputs=evalAionMaskParam(gcb,'value',1)  nOutputs=evalAionMaskParam(gcb,'value',1)  omode=Inherit via internal rule  otype=sfix(16)  scale=2^-15  rndmethod=Unbiased  factor=1  satmethod=Symmetric  shift_vec=[0 1 2 -1]  value=2  inPortNames=[' ' ' ' ' ' ' ' ' ' ' ' ' ' ' ' ' ' ' ' ' ' ' ' ' ' ' ' ' ' ' ' ' ' ' ' ' ' ' ' ' ' ' ' ' ' ' ' ' ' ' ' ' ' ' ' ' ' ' ' ' ' ' ' ' ' ' ' ' ']'  outPortNames=[' ' ' ' ' ' ' ' ' ' ' ' ' ' ' ' ' ' ' ' ' ' ' ' ' ' ' ' ' ' ' ' ' ' ' ' ' ' ' ' ' ' ' ' ' ' ' ' ' ' ' ' ' ' ' ' ' ' ' ' ' ' ' ' ' ' ' ' ' ']'  dspbaimage=dspba_prim.jpg  text=fprintf('GPIn');  style=Optimised  visibilities=1024  latencyCorrection=0  scheduleOrigin=on  version=20090407
  GPOut : DSPBAPrim/GPOut  primtype=gpout  nInputs=evalAionMaskParam(gcb,'value',1)  nOutputs=evalAionMaskParam(gcb,'value',1)  omode=Inherit via internal rule  otype=sfix(16)  scale=2^-15  rndmethod=Unbiased  factor=1  satmethod=Symmetric  shift_vec=[0 1 2 -1]  value=2  inPortNames=[' ' ' ' ' ' ' ' ' ' ' ' ' ' ' ' ' ' ' ' ' ' ' ' ' ' ' ' ' ' ' ' ' ' ' ' ' ' ' ' ' ' ' ' ' ' ' ' ' ' ' ' ' ' ' ' ' ' ' ' ' ' ' ' ' ' ' ' ' ']'  outPortNames=[' ' ' ' ' ' ' ' ' ' ' ' ' ' ' ' ' ' ' ' ' ' ' ' ' ' ' ' ' ' ' ' ' ' ' ' ' ' ' ' ' ' ' ' ' ' ' ' ' ' ' ' ' ' ' ' ' ' ' ' ' ' ' ' ' ' ' ' ' ']'  dspbaimage=dspba_prim.jpg  text=fprintf('GPOut');  style=Optimised  visibilities=1024  latencyCorrection=0  version=20090407
  Sum Of Elements : Subsystem
  SynthesisInfo : DSPBAPrim/SynthesisInfo  primtype=synthinfo  nInputs=0  nOutputs=0  omode=Inherit via internal rule  otype=sfix(16)  scale=2^-15  rndmethod=Truncate  factor=1  satmethod=Symmetric  shift_vec=[0 1 2 -1]  value=99  inPortNames=[' '; ' ';]  outPortNames=[' ']  dspbaimage=dspba_prim_ctrl.jpg  text=fprintf('Style=%s', style);  style=Scheduled  visibilities=2^17+2^18+2^19+2^20  constraintInUse=off  constraintRelation=>  constraintLimit=2  bitAccurate=on  version=20150220
  ^2 : DSPBAPrim/Math  primtype=mathfunc  nInputs=1  nOutputs=1  omode=Inherit via internal rule  otype=sfix(16)  scale=2^-15  rndmethod=Unbiased  factor=1  satmethod=Symmetric  shift_vec=[0 1 2 -1]  value=round([0:255]/17)  inPortNames=[' '; ' ';]  outPortNames=[' ']  dspbaimage=dspba_prim_float.jpg  text=fprintf('exp(x)');  style=Optimised  visibilities=2^17  functionExpr=pow(x;y)  advOptions=[]  floatRounding=correct  version=20130910
  frame_energy_valid : Outport
  frame_eneregy : Outport  Port=2
  wires:
  sample_input/1 -> GPIn/1
  sample_valid/1 -> GPIn/2
  GPOut/1 -> frame_eneregy/1
  ^2/1 -> Sum Of Elements/1(Input)
  GPIn/2 -> Sum Of Elements/2(Valid)
  GPOut/2 -> frame_energy_valid/1
  Sum Of Elements/2(_Valid) -> GPOut/2
  Sum Of Elements/1(Output) -> GPOut/1
  GPIn/1 -> ^2/1
  Const/1 -> ^2/2

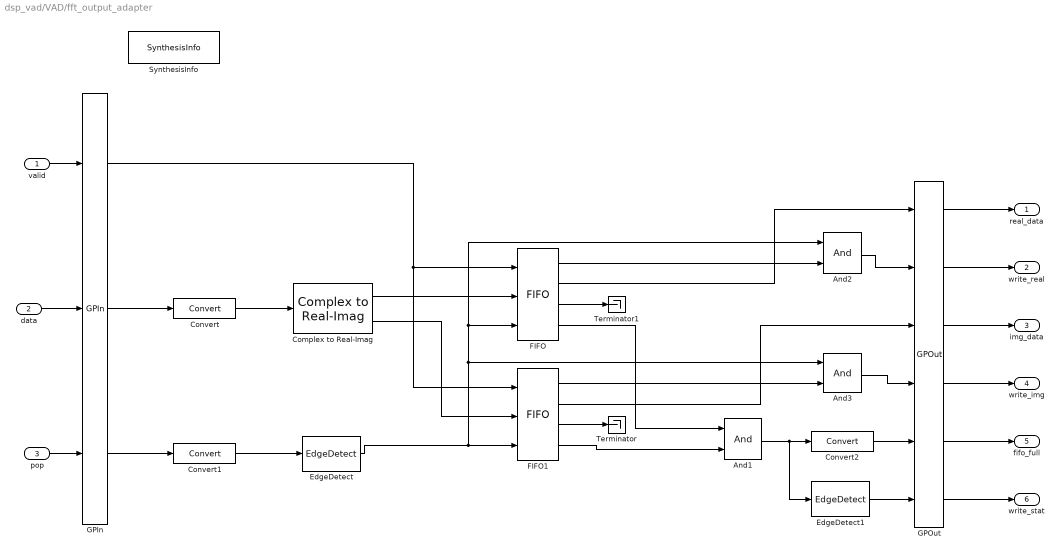
== system dsp_vad/VAD/fft_output_adapter ==
  valid : Inport
  data : Inport  Port=2
  pop : Inport  Port=3
  And1 : DSPBAPrim/And  primtype=and  nInputs=2  nOutputs=1  omode=Inherit via internal rule  otype=sfix(16)  scale=2^-15  rndmethod=Unbiased  factor=1  satmethod=Symmetric  shift_vec=[0 1 2 -1]  value=0  inPortNames=[' '; ' '; ' '; ' '; ' '; ' '; ' '; ' '; ' '; ' '; ' '; ' '; ' '; ' '; ' '; ' '; ]  outPortNames=[' ']  dspbaimage=dspba_prim.jpg  text=fprintf('&');  style=Optimised  visibilities=8+2  version=20090407
  And2 : DSPBAPrim/And  primtype=and  nInputs=2  nOutputs=1  omode=Inherit via internal rule  otype=sfix(16)  scale=2^-15  rndmethod=Unbiased  factor=1  satmethod=Symmetric  shift_vec=[0 1 2 -1]  value=0  inPortNames=[' '; ' '; ' '; ' '; ' '; ' '; ' '; ' '; ' '; ' '; ' '; ' '; ' '; ' '; ' '; ' '; ]  outPortNames=[' ']  dspbaimage=dspba_prim.jpg  text=fprintf('&');  style=Optimised  visibilities=8+2  version=20090407
  And3 : DSPBAPrim/And  primtype=and  nInputs=2  nOutputs=1  omode=Inherit via internal rule  otype=sfix(16)  scale=2^-15  rndmethod=Unbiased  factor=1  satmethod=Symmetric  shift_vec=[0 1 2 -1]  value=0  inPortNames=[' '; ' '; ' '; ' '; ' '; ' '; ' '; ' '; ' '; ' '; ' '; ' '; ' '; ' '; ' '; ' '; ]  outPortNames=[' ']  dspbaimage=dspba_prim.jpg  text=fprintf('&');  style=Optimised  visibilities=8+2  version=20090407
  Complex to Real-Imag : DSPBAVectorUtil/Complex to Real-Imag
  Convert : DSPBAPrim/Convert  primtype=convert  nInputs=1  nOutputs=1  omode=single  otype=sfix(16)  scale=2^-15  rndmethod=Biased  factor=1  satmethod=None  shift_vec=[0 1 2 -1]  value=round([0:255]/17)  inPortNames=[' '; ' ';]  outPortNames=[' '; 'c']  dspbaimage=dspba_prim.jpg  text=fprintf('convert');  style=Optimised  visibilities=8+64+256+2^17  clipdetect=off  floatPrecision=float32_m23  advOptions=[]  version=20130211
  Convert1 : DSPBAPrim/Convert  primtype=convert  nInputs=1  nOutputs=1  omode=boolean  otype=sfix(16)  scale=2^-15  rndmethod=Biased  factor=1  satmethod=None  shift_vec=[0 1 2 -1]  value=round([0:255]/17)  inPortNames=[' '; ' ';]  outPortNames=[' '; 'c']  dspbaimage=dspba_prim.jpg  text=fprintf('convert');  style=Optimised  visibilities=8+64+256+2^17  clipdetect=off  floatPrecision=float32_m23  advOptions=[]  version=20130211
  Convert2 : DSPBAPrim/Convert  primtype=convert  nInputs=1  nOutputs=1  omode=single  otype=sfix(16)  scale=2^-15  rndmethod=Biased  factor=1  satmethod=None  shift_vec=[0 1 2 -1]  value=round([0:255]/17)  inPortNames=[' '; ' ';]  outPortNames=[' '; 'c']  dspbaimage=dspba_prim.jpg  text=fprintf('convert');  style=Optimised  visibilities=8+64+256+2^17  clipdetect=off  floatPrecision=float32_m23  advOptions=[]  version=20130211
  EdgeDetect : DspbAdvFftLibrary/Common/EdgeDetect
  EdgeDetect1 : DspbAdvFftLibrary/Common/EdgeDetect
  FIFO : DSPBAPrim/FIFO  primtype=fifo  nInputs=3  nOutputs=4  omode=Inherit via internal rule  otype=sfix(16)  scale=2^-15  rndmethod=Unbiased  factor=1  satmethod=Symmetric  shift_vec=[0 1 2 -1]  value=[512 1 512]  inPortNames=['w'; 'd'; 'r'; 'f']  outPortNames=['v'; 'q'; 't'; 'f']  dspbaimage=dspba_prim.jpg  text=fprintf('fifo');  style=Optimised  visibilities=263168  version=20130808  user_sclr=off
  FIFO1 : DSPBAPrim/FIFO  primtype=fifo  nInputs=3  nOutputs=4  omode=Inherit via internal rule  otype=sfix(16)  scale=2^-15  rndmethod=Unbiased  factor=1  satmethod=Symmetric  shift_vec=[0 1 2 -1]  value=[512 1 512]  inPortNames=['w'; 'd'; 'r'; 'f']  outPortNames=['v'; 'q'; 't'; 'f']  dspbaimage=dspba_prim.jpg  text=fprintf('fifo');  style=Optimised  visibilities=263168  version=20130808  user_sclr=off
  GPIn : DSPBAPrim/GPIn  primtype=gpin  nInputs=evalAionMaskParam(gcb,'value',1)  nOutputs=evalAionMaskParam(gcb,'value',1)  omode=Inherit via internal rule  otype=sfix(16)  scale=2^-15  rndmethod=Unbiased  factor=1  satmethod=Symmetric  shift_vec=[0 1 2 -1]  value=3  inPortNames=[' ' ' ' ' ' ' ' ' ' ' ' ' ' ' ' ' ' ' ' ' ' ' ' ' ' ' ' ' ' ' ' ' ' ' ' ' ' ' ' ' ' ' ' ' ' ' ' ' ' ' ' ' ' ' ' ' ' ' ' ' ' ' ' ' ' ' ' ' ']'  outPortNames=[' ' ' ' ' ' ' ' ' ' ' ' ' ' ' ' ' ' ' ' ' ' ' ' ' ' ' ' ' ' ' ' ' ' ' ' ' ' ' ' ' ' ' ' ' ' ' ' ' ' ' ' ' ' ' ' ' ' ' ' ' ' ' ' ' ' ' ' ' ']'  dspbaimage=dspba_prim.jpg  text=fprintf('GPIn');  style=Optimised  visibilities=1024  latencyCorrection=0  scheduleOrigin=on  version=20090407
  GPOut : DSPBAPrim/GPOut  primtype=gpout  nInputs=evalAionMaskParam(gcb,'value',1)  nOutputs=evalAionMaskParam(gcb,'value',1)  omode=Inherit via internal rule  otype=sfix(16)  scale=2^-15  rndmethod=Unbiased  factor=1  satmethod=Symmetric  shift_vec=[0 1 2 -1]  value=6  inPortNames=[' ' ' ' ' ' ' ' ' ' ' ' ' ' ' ' ' ' ' ' ' ' ' ' ' ' ' ' ' ' ' ' ' ' ' ' ' ' ' ' ' ' ' ' ' ' ' ' ' ' ' ' ' ' ' ' ' ' ' ' ' ' ' ' ' ' ' ' ' ']'  outPortNames=[' ' ' ' ' ' ' ' ' ' ' ' ' ' ' ' ' ' ' ' ' ' ' ' ' ' ' ' ' ' ' ' ' ' ' ' ' ' ' ' ' ' ' ' ' ' ' ' ' ' ' ' ' ' ' ' ' ' ' ' ' ' ' ' ' ' ' ' ' ']'  dspbaimage=dspba_prim.jpg  text=fprintf('GPOut');  style=Optimised  visibilities=1024  latencyCorrection=0  version=20090407
  SynthesisInfo : DSPBAPrim/SynthesisInfo  primtype=synthinfo  nInputs=0  nOutputs=0  omode=Inherit via internal rule  otype=sfix(16)  scale=2^-15  rndmethod=Truncate  factor=1  satmethod=Symmetric  shift_vec=[0 1 2 -1]  value=99  inPortNames=[' '; ' ';]  outPortNames=[' ']  dspbaimage=dspba_prim_ctrl.jpg  text=fprintf('Style=%s', style);  style=Scheduled  visibilities=2^17+2^18+2^19+2^20  constraintInUse=off  constraintRelation=>  constraintLimit=2  bitAccurate=on  version=20150220
  Terminator : Terminator
  Terminator1 : Terminator
  real_data : Outport
  write_real : Outport  Port=2
  img_data : Outport  Port=3
  write_img : Outport  Port=4
  fifo_full : Outport  Port=5
  write_stat : Outport  Port=6
  wires:
  Complex to Real-Imag/2 -> FIFO1/2
  FIFO1/3 -> Terminator/1
  FIFO/3 -> Terminator1/1
  FIFO/4 -> And1/1
  FIFO1/4 -> And1/2
  And1/1 -> EdgeDetect1/1, Convert2/1
  valid/1 -> GPIn/1
  data/1 -> GPIn/2
  pop/1 -> GPIn/3
  GPIn/3 -> Convert1/1
  GPIn/1 -> FIFO1/1, FIFO/1
  Convert1/1 -> EdgeDetect/1
  GPIn/2 -> Convert/1
  GPOut/1 -> real_data/1
  GPOut/3 -> img_data/1
  GPOut/2 -> write_real/1
  GPOut/4 -> write_img/1
  GPOut/5 -> fifo_full/1
  GPOut/6 -> write_stat/1
  FIFO/1 -> And2/2
  Convert2/1 -> GPOut/5
  EdgeDetect/1 -> And2/1, FIFO/3, And3/1, FIFO1/3
  EdgeDetect1/1 -> GPOut/6
  FIFO/2 -> GPOut/1
  And2/1 -> GPOut/2
  FIFO1/1 -> And3/2
  And3/1 -> GPOut/4
  FIFO1/2 -> GPOut/3
  Complex to Real-Imag/1 -> FIFO/2
  Convert/1 -> Complex to Real-Imag/1
